simulink subsystem "FCS_Out"  (R2025a)
settings: Solver=VariableStepAuto  StartTime=0.0  StopTime=10.0  RelTol=1e-3
settings Model: Creator=gurt1  LastModifiedBy=gurt1

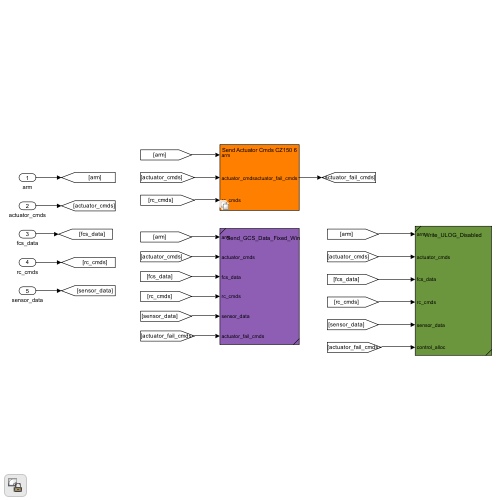
[thumbnail: Simulink's stored preview of the top-level diagram]
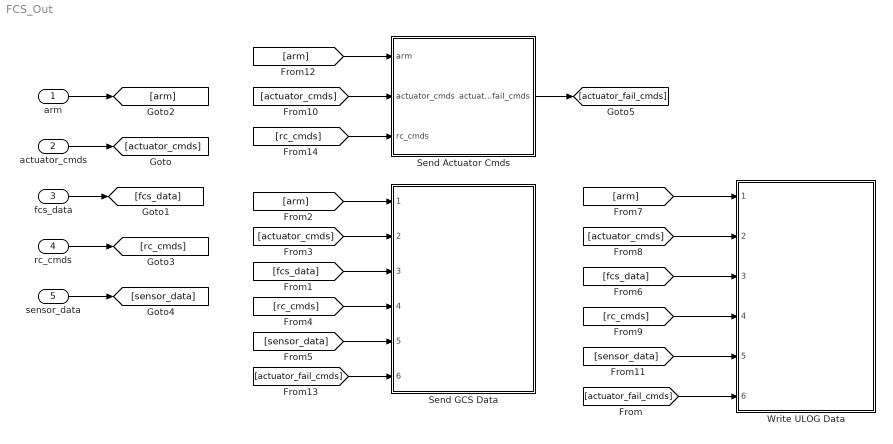
== system FCS_Out ==
  arm : Inport
  actuator_cmds : Inport  Port=2
  fcs_data : Inport  Port=3
  rc_cmds : Inport  Port=4
  sensor_data : Inport  Port=5
  Send Actuator Cmds : Subsystem  Variant=on  EmptyChoice=on
  Send GCS Data : Subsystem  ReferencedSubsystem=Send_GCS_Data_Fixed_Wing
  Write ULOG Data : Subsystem  ReferencedSubsystem=Write_ULOG_Data
  wires:
  actuator_cmds/1 -> [actuator_cmds]
  fcs_data/1 -> [fcs_data]
  arm/1 -> [arm]
  rc_cmds/1 -> [rc_cmds]
  sensor_data/1 -> [sensor_data]
  [arm] -> Write ULOG Data/1
  [actuator_cmds] -> Write ULOG Data/2
  [fcs_data] -> Write ULOG Data/3
  [rc_cmds] -> Write ULOG Data/4
  [sensor_data] -> Write ULOG Data/5
  [arm] -> Send GCS Data/1
  [actuator_cmds] -> Send GCS Data/2
  [fcs_data] -> Send GCS Data/3
  [rc_cmds] -> Send GCS Data/4
  [sensor_data] -> Send GCS Data/5
  [actuator_fail_cmds] -> Write ULOG Data/6
  [actuator_fail_cmds] -> Send GCS Data/6
  [arm] -> Send Actuator Cmds/1(arm)
  [actuator_cmds] -> Send Actuator Cmds/2(actuator_cmds)
  [rc_cmds] -> Send Actuator Cmds/3(rc_cmds)
  Send Actuator Cmds/1(actuator_fail_cmds) -> [actuator_fail_cmds]

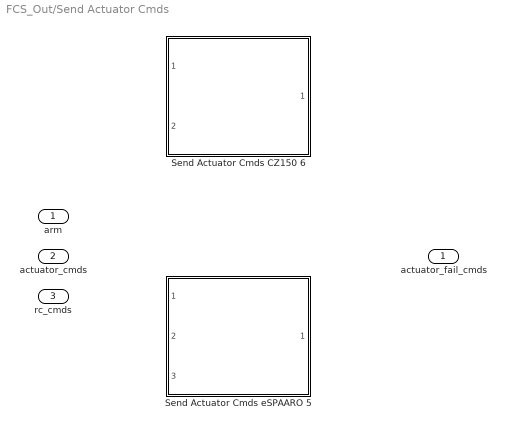
== system FCS_Out/Send Actuator Cmds ==
  arm : Inport
  actuator_cmds : Inport  Port=2
  rc_cmds : Inport  Port=3
  Send Actuator Cmds CZ150 6 : Subsystem  VariantControl=FW_type == 1  ReferencedSubsystem=Send_Actuator_Cmds_CZ1506
  Send Actuator Cmds eSPAARO 5 : Subsystem  VariantControl=FW_type == 2  ReferencedSubsystem=Send_Actuator_Cmds_eSPAARO5
  actuator_fail_cmds : Outport
